simulink model "Motor_einfaches_modell"  (Simulink 7.1)
settings: Solver=ode45  StartTime=0  StopTime=2  FixedStep=0.01  MaxStep=0.01  RelTol=1e-3
undefined symbols (not defined in the file): Ispez, J, L, R
settings Model: Creator=dep19025415  LastModifiedBy=dep19025415

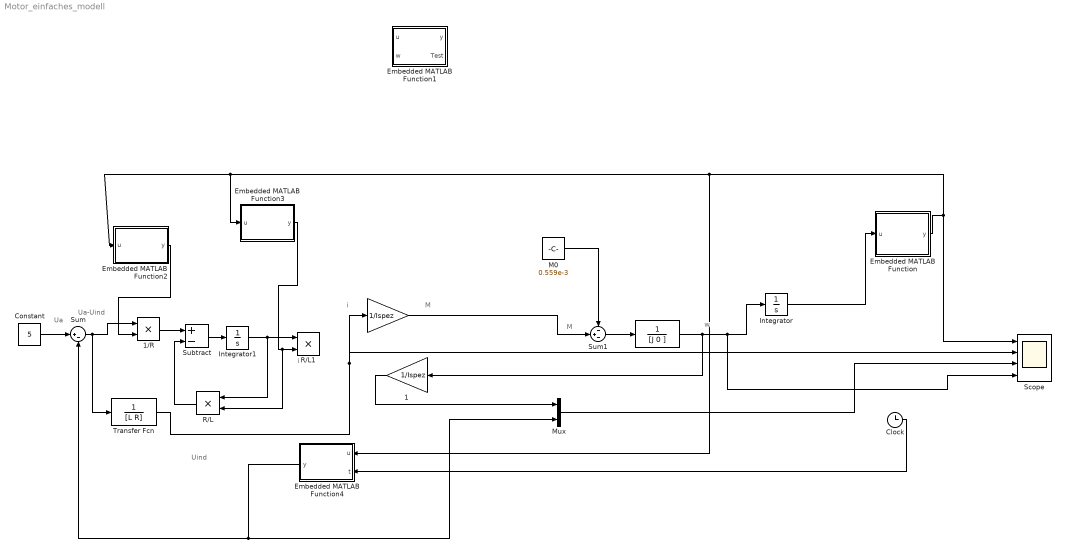
== system Motor_einfaches_modell ==
  note: Uind
  note: Ua-Uind
  note: i
  note: M
  note: w
  note: Ua
  note: i
  note: M
  " " : Gain  Gain=1/Ispez  ParameterDataType=sfix(16)  ParameterScaling=2^0  OutDataType=sfix(16)  OutScaling=2^0
  "      " : TransferFcn  Denominator=[J 0 ]
  " 1" : Gain  Orientation=left  Gain=1/Ispez  ParameterDataType=sfix(16)  ParameterScaling=2^0  OutDataType=sfix(16)  OutScaling=2^0
  1/R : Product  OutDataType=sfix(16)  OutScaling=2^0  RndMeth=Zero
  Clock : Clock
      settings: Decimation=10
  Constant : Constant  Value=5  OutDataType=sfix(16)  OutScaling=2^0
  Embedded MATLAB Function : Stateflow chart
  Embedded MATLAB Function1 : Stateflow chart
  Embedded MATLAB Function2 : Stateflow chart
  Embedded MATLAB Function3 : Stateflow chart
  Embedded MATLAB Function4 : Stateflow chart  Orientation=left
  Integrator : Integrator
  Integrator1 : Integrator
  M0 : Constant  Value=0.559e-3  OutDataType=sfix(16)  OutScaling=2^0
  Mux : Mux  Inputs=2
  R/L : Product  Orientation=left  OutDataType=sfix(16)  OutScaling=2^0  RndMeth=Zero
  R/L1 : Product  OutDataType=sfix(16)  OutScaling=2^0  RndMeth=Zero
  Scope : Scope  NumInputPorts=4
      settings: YMin=0~0.1125~2.5~900  YMax=375~0.1275~30~2000
  Subtract : Sum  Inputs=+-  OutDataType=sfix(16)  OutScaling=2^-10
  Sum : Sum  Inputs=|+-  OutDataType=sfix(16)  OutScaling=2^0
  Sum1 : Sum  Inputs=-+-  OutDataType=sfix(16)  OutScaling=2^0
  Transfer Fcn : TransferFcn  Denominator=[L R]
  wires:
  Sum1/1 -> "      "/1
  Constant/1 -> Sum/1
  "      "/1 -> " 1"/1, Integrator/1, Scope/4
  Integrator/1 -> Embedded MATLAB Function/1(u)
  Embedded MATLAB Function/1(y) -> Scope/1, Embedded MATLAB Function3/1(u), Embedded MATLAB Function2/1(u), Embedded MATLAB Function4/1(u)
  Subtract/1 -> Integrator1/1
  Integrator1/1 -> R/L/1, R/L1/1
  R/L/1 -> Subtract/2
  1/R/1 -> Subtract/1
  Embedded MATLAB Function2/1(y) -> 1/R/2
  Embedded MATLAB Function3/1(y) -> R/L1/2, R/L/2
  " "/1 -> Sum1/2
  Sum/1 -> 1/R/1, Transfer Fcn/1
  Clock/1 -> Embedded MATLAB Function4/2(t)
  Embedded MATLAB Function4/1(y) -> Sum/2, Mux/2
  " 1"/1 -> Mux/1
  Mux/1 -> Scope/3
  Transfer Fcn/1 -> " "/1, Scope/2
  M0/1 -> Sum1/1

== matlab function Embedded MATLAB Function1 ==
  data: u input double; y output double; w input double; Test output double
function [y,Test] = fcn(u, w)
%function y = fcn(u)
% This block supports the Embedded MATLAB subset.
% See the help menu for details. 


%y = u;
y = nan;
Test = 0;
y = u;
if (w > 0 && w <0.1) || (w > 120 && w < 121.1) || (w > 240 && w < 241.1)  
    y = u * (2/3);
    Test = 1;
end

end

== matlab function Embedded MATLAB Function ==
  data: u input double; y output double
function y = fcn(u)
%function y = fcn(u)
% This block supports the Embedded MATLAB subset.
% See the help menu for details. 



%eml.extrinsic('save_to_base')

y = u;

% if u >= ((Run) * 360) && u < ((Run + 1)*360)
%    Run = Run + 1;
%   % save_to_base(Run);
%   data = Run;
% end
% 
% y = u - ((Run-1) * 360);

if u >= 360 && u <=720
    y= u-360;
end
if u >= 720 && u <=1080
    y= u-720;
end
if u >= 1080 && u <=1440
    y= u-1080;
end
if u >= 1440 && u <=1800
    y= u-1440;
end
if u >= 1800 && u <=2160
    y= u-1800;
end
if u >= 2160 && u <=2520
    y= u-2160;
end
if u >= 2520 && u <=2880
    y= u-2520;
end
if u >= 2880 && u <=3240
    y= u-2880;
end






    
    

end

== matlab function Embedded MATLAB Function2 ==
  data: u input double; y output double
function y = fcn(u)
% This block supports the Embedded MATLAB subset.
% See the help menu for details. 

y = (1/9.1);
if (u > 0 && u <1) || (u > 120 && u < 121) || (u > 240 && u < 241)  
   y = (1/6.825); 
end

end

== matlab function Embedded MATLAB Function3 ==
  data: u input double; y output double
function y = fcn(u)
% This block supports the Embedded MATLAB subset.
% See the help menu for details. 


y = (9.1/7.4e-3);
if (u > 0 && u <3) || (u > 120 && u < 123) || (u > 240 && u < 243)  
   y = (6.825/5.5e-3); 
end

end

== matlab function Embedded MATLAB Function4 ==
  data: u input double; y output double; t input double
function y = fcn(u, t)
% This block supports the Embedded MATLAB subset.
% See the help menu for details. 

y = nan;
x=0;
for m=1:1:1000
    x = x + ((cos(6*m*u*pi/180))/(36*m*m-1)); 
end
    y = (6/pi) * 4.42 * (1/2 - x);
%y=u*1/58;


end
